simulink model "Sim_NL_XZ"  (R2016a)
settings: Solver=FixedStepAuto  SolverMode=SingleTasking  StartTime=0.0  StopTime=2  RelTol=1e-3
libraries: simulink x1
settings Model: Creator=Florian  LastModifiedBy=Florian
settings OptimizationCC: DefaultParameterBehavior=Inlined  UseDivisionForNetSlopeComputation=on  UseFloatMulNetSlope=on  InlineInvariantSignals=on  PassReuseOutputArgsAs=Individual arguments  ZeroExternalMemoryAtStartup=off  ZeroInternalMemoryAtStartup=off  NoFixptDivByZeroProtection=on  EfficientFloat2IntCast=on  OptimizeModelRefInitCode=on  LifeSpan=1
settings HardwareCC: ProdBitPerPointer=32  ProdLargestAtomicInteger=Long  ProdLargestAtomicFloat=Double  ProdWordSize=32  ProdHWDeviceType=ARM Compatible->ARM Cortex
settings RTWCC: SystemTargetFile=ert.tlc  TemplateMakefile=ert_default_tmf  GenerateReport=on  IncludeHyperlinkInReport=on  LaunchReport=on  GenerateTraceInfo=on  GenerateTraceReport=on  GenerateTraceReportSl=on  GenerateTraceReportSf=on  GenerateTraceReportEml=on  GenerateCodeMetricsReport=on
settings CodeAppCC: ForceParamTrailComments=on  IgnoreCustomStorageClasses=off  OperatorAnnotations=on  SimulinkDataObjDesc=on  SFDataObjDesc=on  MATLABFcnDesc=on  InsertBlockDesc=on  MATLABSourceComments=on
settings ERTTargetCC: GenerateSampleERTMain=on  IncludeMdlTerminateFcn=off  CombineSignalStateStructs=on  SupportComplex=off  SupportContinuousTime=on  InlinedParameterPlacement=NonHierarchical  ERTCustomFileTemplate=example_file_process.tlc  ERTFilePackagingFormat=CompactWithDataFile

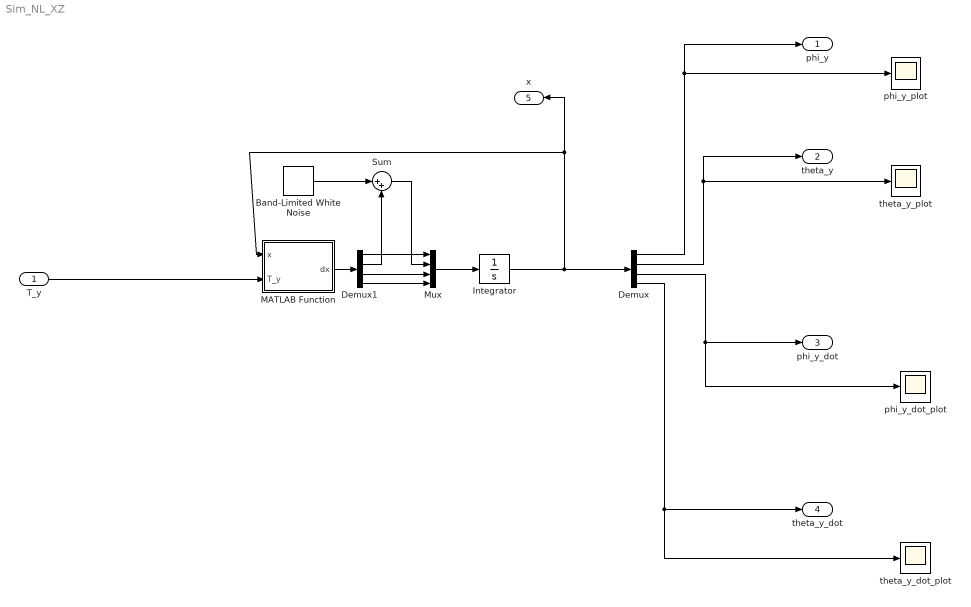
== system Sim_NL_XZ ==
  "T_y " : Inport
  Band-Limited White Noise : simulink/Sources/Band-Limited White Noise  Cov=[0.1^2]  Ts=1/92  seed=[23341]
  Demux : Demux
  Demux1 : Demux
  Integrator : Integrator  InitialCondition="[0 pi/32  0 0]"
  MATLAB Function : MATLAB Function  TreatAsAtomicUnit=on
  Mux : Mux
  Sum : Sum  Inputs=|++
  phi_y_dot_plot : Scope
  phi_y_plot : Scope
  theta_y_dot_plot : Scope
  theta_y_plot : Scope
  phi_y : Outport
  theta_y : Outport  Port=2
  phi_y_dot : Outport  Port=3
  theta_y_dot : Outport  Port=4
  x : Outport  Port=5
  wires:
  Integrator/1 -> x/1, MATLAB Function/1(x), Demux/1
  Demux/1 -> phi_y_plot/1, phi_y/1
  Demux/2 -> theta_y/1, theta_y_plot/1
  Demux/3 -> phi_y_dot_plot/1, phi_y_dot/1
  Demux/4 -> theta_y_dot_plot/1, theta_y_dot/1
  "T_y "/1 -> MATLAB Function/2(T_y)
  MATLAB Function/1(dx) -> Demux1/1
  Demux1/1 -> Mux/1
  Mux/1 -> Integrator/1
  Demux1/2 -> Sum/2
  Sum/1 -> Mux/2
  Demux1/3 -> Mux/3
  Demux1/4 -> Mux/4
  Band-Limited White Noise/1 -> Sum/1

== matlab function Sim_NL_XZ/MATLAB Function ==
  data: x input; T_y input; dx output
function dx = fcn_xz(x,T_y)

%Zuweisung Koordinaten und Ableitungen
phi_y =x(1);
theta_y=x(2);
phi_y_dot=x(3);
theta_y_dot=x(4);

phi_y_dotdot =(0.0355556*(1.65925e33*sin(theta_y)*theta_y_dot^2 + 5.804e34*T_y + 1.26585e35*sin(theta_y) - 8.4019e33*cos(theta_y)*sin(theta_y) + 4.60272e33*T_y*cos(theta_y)))/(6.42314e31*cos(theta_y) - 2.13164e30*cos(theta_y)^2 + 1.63981e32);

theta_y_dotdot = (0.111111*(6.01665e33*T_y + 2.95242e34*sin(theta_y) + 2.89041e32*theta_y_dot^2*sin(theta_y) - 1.47287e33*T_y*cos(theta_y) - 1.91848e31*theta_y_dot^2*cos(theta_y)*sin(theta_y)))/(6.42314e31*cos(theta_y) - 2.13164e30*cos(theta_y)^2 + 1.63981e32);

%Zuweisung Ausgang
dx = [phi_y_dot; theta_y_dot; phi_y_dotdot; theta_y_dotdot];
end
